simulink model "guid_full_loop_no_rot"  (R2021a)
settings: Solver=VariableStepAuto  StartTime=0.0  StopTime=5  RelTol=1e-3
values from neighbouring files (symbols this model uses):
  Ahg3 = blkdiag(Ahg3, Ahcg)    [ranger_full_indi_sim.m]
  Bhg3 = blkdiag(Bhg3, Bhcg)    [ranger_full_indi_sim.m]
  Chg3 = blkdiag(Chg3, Chcg)    [ranger_full_indi_sim.m]
  Dhg3 = blkdiag(Dhg3, Dhcg)    [ranger_full_indi_sim.m]
  Kdg = [2.0; 2.0; 1.8]    [ranger_full_indi_sim.m]
  Kpg = [0.581; 0.581; 0.5943]    [ranger_full_indi_sim.m]
settings Model: Creator=AutomZ2-RG02B04  LastModifiedBy=AutomZ2-RG02A02
settings SolverCC: AlgebraicLoopSolver=TrustRegion

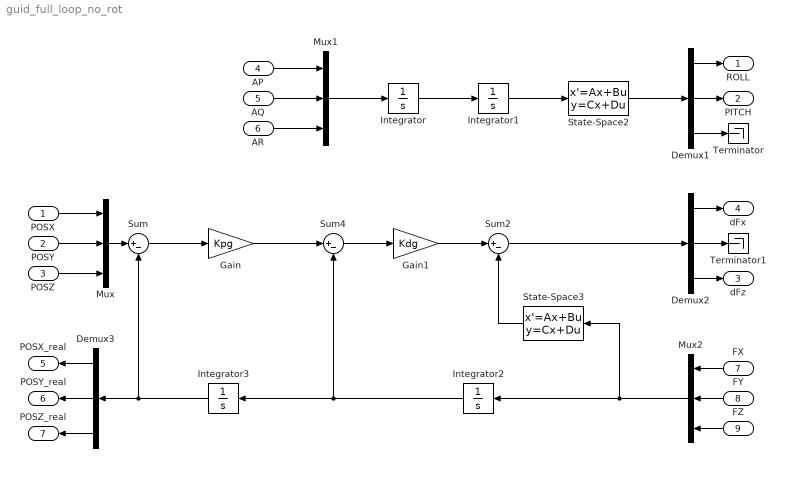
== system guid_full_loop_no_rot ==
  POSX : Inport
  POSY : Inport  Port=2
  POSZ : Inport  Port=3
  AP : Inport  Port=4
  AQ : Inport  Port=5
  AR : Inport  Port=6
  FX : Inport  Port=7
  FY : Inport  Port=8
  FZ : Inport  Port=9
  Demux1 : Demux  Outputs=3
  Demux2 : Demux  Outputs=3
  Demux3 : Demux  Outputs=3
  Gain : Gain  Gain=Kpg
  Gain1 : Gain  Gain=Kdg
  Integrator{,1..3} (4 alike) : Integrator
  Mux : Mux  Inputs=3
  Mux1 : Mux  Inputs=3
  Mux2 : Mux  Inputs=3
  State-Space2 : StateSpace  A=Ahg3  B=Bhg3  C=Chg3  D=Dhg3  InitialCondition=0
  State-Space3 : StateSpace  A=Ahg3  B=Bhg3  C=Chg3  D=Dhg3  InitialCondition=0
  Sum : Sum  Inputs=|+-
  Sum2 : Sum  Inputs=|+-
  Sum4 : Sum  Inputs=|+-
  Terminator : Terminator
  Terminator1 : Terminator
  ROLL : Outport
  PITCH : Outport  Port=2
  dFz : Outport  Port=3
  dFx : Outport  Port=4
  POSX_real : Outport  Port=5
  POSY_real : Outport  Port=6
  POSZ_real : Outport  Port=7
  wires:
  Sum/1 -> Gain/1
  POSY/1 -> Mux/2
  POSZ/1 -> Mux/3
  Mux/1 -> Sum/1
  Demux2/1 -> dFx/1
  POSX/1 -> Mux/1
  Gain/1 -> Sum4/1
  Sum4/1 -> Gain1/1
  Gain1/1 -> Sum2/1
  AP/1 -> Mux1/1
  AQ/1 -> Mux1/2
  AR/1 -> Mux1/3
  Mux1/1 -> Integrator/1
  Mux2/1 -> Integrator2/1, State-Space3/1
  Integrator/1 -> Integrator1/1
  Integrator1/1 -> State-Space2/1
  State-Space2/1 -> Demux1/1
  Demux1/3 -> Terminator/1
  Demux1/1 -> ROLL/1
  Demux1/2 -> PITCH/1
  FX/1 -> Mux2/1
  FY/1 -> Mux2/2
  Integrator2/1 -> Sum4/2, Integrator3/1
  Integrator3/1 -> Demux3/1, Sum/2
  FZ/1 -> Mux2/3
  State-Space3/1 -> Sum2/2
  Sum2/1 -> Demux2/1
  Demux2/3 -> dFz/1
  Demux2/2 -> Terminator1/1
  Demux3/1 -> POSX_real/1
  Demux3/2 -> POSY_real/1
  Demux3/3 -> POSZ_real/1
